simulink model "mainModel"  (R2025a)
settings: Solver=VariableStepAuto  StartTime=0  StopTime=5000  RelTol=1e-3
values from neighbouring files (symbols this model uses):
  advectiveCoefficientScale = 400    [constant_parameters.m]    (also in runScript.m = 100)
  AmbientTemperature = out{4}    [runScript.m]
  massCoolantScale = 0.01    [constant_parameters.m]    (also in runScript.m = 0.003)
  massModuleScale = 11    [constant_parameters.m]    (also in runScript.m)
  scaledAdvectiveCoefficient = 1.2    [runScript.m]
  scaledMassCoolant = 0.8    [runScript.m]
  scaledMassModule = 1.2    [runScript.m]
libraries: fl_lib x231, coolantFlow_lib x65, nesl_utility x35, IONIQ_parameters2_lib x32, algebraicManip_lib x32, batt_lib x1
settings Model: Creator=mbhattu  LastModifiedBy=mbhattu
settings SimscapeCC: SimscapeLogType=all

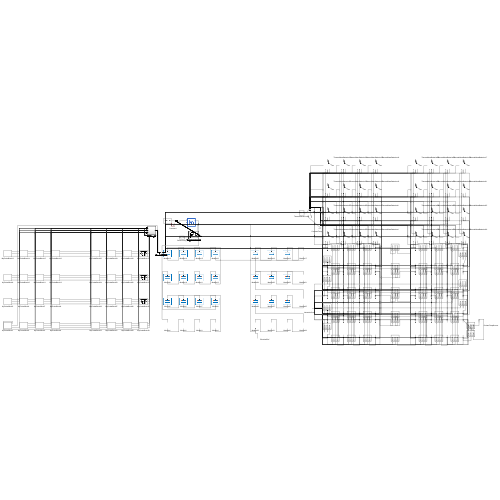
[thumbnail: Simulink's stored preview of the top-level diagram]
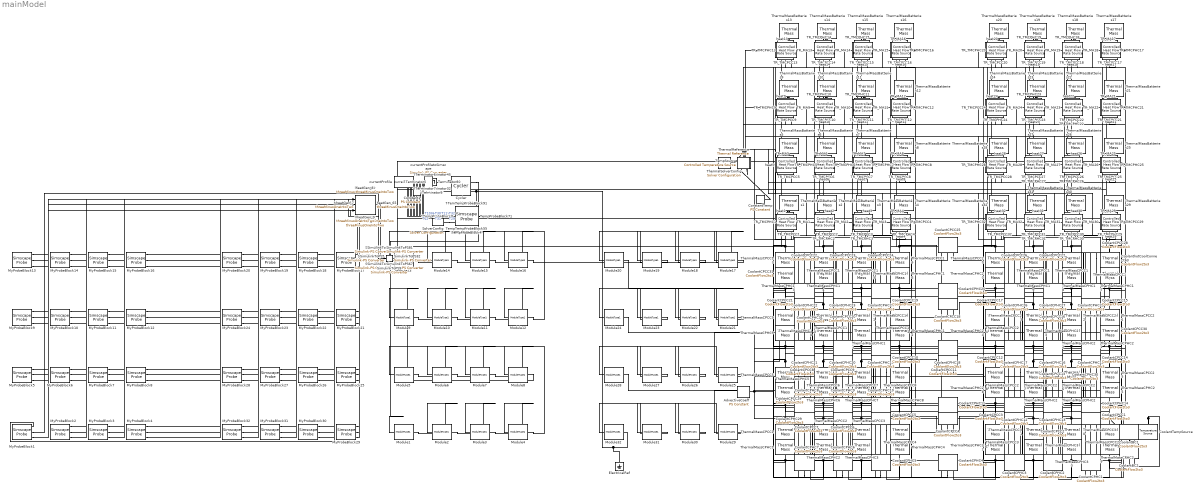
== system mainModel ==
  AdvectiveCoeff : fl_lib/Physical Signals/Sources/PS Constant  constant=advectiveCoefficientScale * scaledAdvectiveCoefficient W/K
  Constant1 : fl_lib/Physical Signals/Sources/PS Constant  constant=1
  ConstantTemp : fl_lib/Physical Signals/Sources/PS Constant  constant=AmbientTemperature
  CoolantBC1 : coolantFlow_lib/CoolantFlow2to3  SystemSampleTime=-1  VariantActivationTime=update diagram  EmptyChoice=off  PassThrough=off  PassThroughVariantControl=(default)  EmptyChoiceVariantControl=(default)  AllowFlexibleInterface=on  Latency=0  AutoFrameSizeCalculation=off
  CoolantBC2 : coolantFlow_lib/CoolantFlow2to3  SystemSampleTime=-1  VariantActivationTime=update diagram  EmptyChoice=off  PassThrough=off  PassThroughVariantControl=(default)  EmptyChoiceVariantControl=(default)  AllowFlexibleInterface=on  Latency=0  AutoFrameSizeCalculation=off
  CoolantCPCC{1..31} (31 alike) : coolantFlow_lib/CoolantFlow2to3  SystemSampleTime=-1  VariantActivationTime=update diagram  EmptyChoice=off  PassThrough=off  PassThroughVariantControl=(default)  EmptyChoiceVariantControl=(default)  AllowFlexibleInterface=on  Latency=0  AutoFrameSizeCalculation=off
  CoolantCPHC{1..31} (31 alike) : coolantFlow_lib/CoolantFlow2to3  SystemSampleTime=-1  VariantActivationTime=update diagram  EmptyChoice=off  PassThrough=off  PassThroughVariantControl=(default)  EmptyChoiceVariantControl=(default)  AllowFlexibleInterface=on  Latency=0  AutoFrameSizeCalculation=off
  CoolantTempSource : fl_lib/Thermal/Thermal Sources/Temperature Source  temperature=coolantTempSourceTemperature K
  CoolanthotCoolConnect63 : coolantFlow_lib/CoolantFlow2to3  SystemSampleTime=-1  VariantActivationTime=update diagram  EmptyChoice=off  PassThrough=off  PassThroughVariantControl=(default)  EmptyChoiceVariantControl=(default)  AllowFlexibleInterface=on  Latency=0  AutoFrameSizeCalculation=off
  Cycler : batt_lib/Cyclers/Cycler  current_option=simscape.battery.enum.cyclers.positive_current.Discharge  configuration_option=simscape.battery.enum.cyclers.device_configuration.Cycler
      settings: InternalSimscapePortConfiguration="{\"Bottom\":[],\"Left\":[{\"id\":\"iT\",\"label\":\"i\",\"type\":\"input\"},{\"id\":\"vT\",\"label\":\"v\",\"type\":\"input\"},{\"id\":\"c\",\"label\":\"c\",\"type\":\"input\"}],\"Right\":[{\"id\":\"p\",\"label\":\"+\",\"type\":\"foundation.electrical.electrical\"},{\"id\":\"n\",\"label\":\"-\",\"type\":\"foundation.electrical.electrical\"}],\"Top\":[]}"
  ElectricalRef : fl_lib/Electrical/Electrical Elements/Electrical Reference
  Module{1..32} (32 alike) : IONIQ_parameters2_lib/Modules/ModuleType1  BatteryCapacityCell=ModuleType1.BatteryCapacityCell A*hr  ExtrapolationMethodCell=simscape.enum.extrapolation.nearest  SOCBreakpointsCell=ModuleType1.SOCBreakpointsCell  TemperatureBreakpointsCell=ModuleType1.TemperatureBreakpointsCell K  OpenCircuitVoltageThermalCell=ModuleType1.OpenCircuitVoltageThermalCell V  VoltageRangeCell=ModuleType1.VoltageRangeCell V  ResistanceSOCBreakpointsCell=ModuleType1.ResistanceSOCBreakpointsCell  ResistanceTemperatureBreakpointsCell=ModuleType1.ResistanceTemperatureBreakpointsCell K  R0ThermalCell=ModuleType1.R0ThermalCell Ohm  R1ThermalCell=ModuleType1.R1ThermalCell Ohm  Tau1ThermalCell=ModuleType1.Tau1ThermalCell s  SimulationTemperatureCell=ModuleType1.SimulationTemperatureCell K  P=2  S=6  socCell_specify=on  socCell_priority=High  socCell=Module1.socCell  socCell_nominal_specify=off  socCell_nominal_value=1  socCell_nominal_unit=1  batteryVoltage_specify=on  batteryVoltage_priority=None  batteryVoltage=Module1.batteryVoltage V  batteryVoltage_nominal_specify=off  batteryVoltage_nominal_value=1  batteryVoltage_nominal_unit=V  batteryCurrent_specify=on  batteryCurrent_priority=None  batteryCurrent=Module1.batteryCurrent A  batteryCurrent_nominal_specify=off  batteryCurrent_nominal_value=1  batteryCurrent_nominal_unit=A  numCycles_specify=on  numCycles_priority=High  numCycles=Module1.numCycles  numCycles_nominal_specify=off  numCycles_nominal_value=1  numCycles_nominal_unit=1  vParallelAssembly_specify=on  vParallelAssembly_priority=None  vParallelAssembly=Module1.vParallelAssembly V  vParallelAssembly_nominal_specify=off  vParallelAssembly_nominal_value=1  vParallelAssembly_nominal_unit=V  socParallelAssembly_specify=on  socParallelAssembly_priority=None  socParallelAssembly=Module1.socParallelAssembly  socParallelAssembly_nominal_specify=off  socParallelAssembly_nominal_value=1  socParallelAssembly_nominal_unit=1
      settings: InternalSimscapePortConfiguration="{\"Bottom\":[{\"id\":\"n\",\"label\":\"-\",\"type\":\"foundation.electrical.electrical\"}],\"Left\":[],\"Right\":[],\"Top\":[{\"id\":\"p\",\"label\":\"+\",\"type\":\"foundation.electrical.electrical\"}]}"
  MyProbeBlock1 : SimscapeProbe  BoundBlock=1  Variables="{\"Cell1.batteryCurrent\":{\"Probing\":\"ON\"},\"Cell1.batteryVoltage\":{\"Probing\":\"ON\"},\"Cell1.ocv\":{\"Probing\":\"ON\"}}"
  MyProbeBlock10 : SimscapeProbe  BoundBlock=10  Variables="{\"Cell1.batteryCurrent\":{\"Probing\":\"ON\"},\"Cell1.batteryVoltage\":{\"Probing\":\"ON\"},\"Cell1.ocv\":{\"Probing\":\"ON\"}}"
  MyProbeBlock11 : SimscapeProbe  BoundBlock=11  Variables="{\"Cell1.batteryCurrent\":{\"Probing\":\"ON\"},\"Cell1.batteryVoltage\":{\"Probing\":\"ON\"},\"Cell1.ocv\":{\"Probing\":\"ON\"}}"
  MyProbeBlock12 : SimscapeProbe  BoundBlock=12  Variables="{\"Cell1.batteryCurrent\":{\"Probing\":\"ON\"},\"Cell1.batteryVoltage\":{\"Probing\":\"ON\"},\"Cell1.ocv\":{\"Probing\":\"ON\"}}"
  MyProbeBlock13 : SimscapeProbe  BoundBlock=13  Variables="{\"Cell1.batteryCurrent\":{\"Probing\":\"ON\"},\"Cell1.batteryVoltage\":{\"Probing\":\"ON\"},\"Cell1.ocv\":{\"Probing\":\"ON\"}}"
  MyProbeBlock14 : SimscapeProbe  BoundBlock=14  Variables="{\"Cell1.batteryCurrent\":{\"Probing\":\"ON\"},\"Cell1.batteryVoltage\":{\"Probing\":\"ON\"},\"Cell1.ocv\":{\"Probing\":\"ON\"}}"
  MyProbeBlock15 : SimscapeProbe  BoundBlock=15  Variables="{\"Cell1.batteryCurrent\":{\"Probing\":\"ON\"},\"Cell1.batteryVoltage\":{\"Probing\":\"ON\"},\"Cell1.ocv\":{\"Probing\":\"ON\"}}"
  MyProbeBlock16 : SimscapeProbe  BoundBlock=16  Variables="{\"Cell1.batteryCurrent\":{\"Probing\":\"ON\"},\"Cell1.batteryVoltage\":{\"Probing\":\"ON\"},\"Cell1.ocv\":{\"Probing\":\"ON\"}}"
  MyProbeBlock17 : SimscapeProbe  BoundBlock=17  Variables="{\"Cell1.batteryCurrent\":{\"Probing\":\"ON\"},\"Cell1.batteryVoltage\":{\"Probing\":\"ON\"},\"Cell1.ocv\":{\"Probing\":\"ON\"}}"
  MyProbeBlock18 : SimscapeProbe  BoundBlock=18  Variables="{\"Cell1.batteryCurrent\":{\"Probing\":\"ON\"},\"Cell1.batteryVoltage\":{\"Probing\":\"ON\"},\"Cell1.ocv\":{\"Probing\":\"ON\"}}"
  MyProbeBlock19 : SimscapeProbe  BoundBlock=19  Variables="{\"Cell1.batteryCurrent\":{\"Probing\":\"ON\"},\"Cell1.batteryVoltage\":{\"Probing\":\"ON\"},\"Cell1.ocv\":{\"Probing\":\"ON\"}}"
  MyProbeBlock2 : SimscapeProbe  BoundBlock=2  Variables="{\"Cell1.batteryCurrent\":{\"Probing\":\"ON\"},\"Cell1.batteryVoltage\":{\"Probing\":\"ON\"},\"Cell1.ocv\":{\"Probing\":\"ON\"}}"
  MyProbeBlock20 : SimscapeProbe  BoundBlock=20  Variables="{\"Cell1.batteryCurrent\":{\"Probing\":\"ON\"},\"Cell1.batteryVoltage\":{\"Probing\":\"ON\"},\"Cell1.ocv\":{\"Probing\":\"ON\"}}"
  MyProbeBlock21 : SimscapeProbe  BoundBlock=21  Variables="{\"Cell1.batteryCurrent\":{\"Probing\":\"ON\"},\"Cell1.batteryVoltage\":{\"Probing\":\"ON\"},\"Cell1.ocv\":{\"Probing\":\"ON\"}}"
  MyProbeBlock22 : SimscapeProbe  BoundBlock=22  Variables="{\"Cell1.batteryCurrent\":{\"Probing\":\"ON\"},\"Cell1.batteryVoltage\":{\"Probing\":\"ON\"},\"Cell1.ocv\":{\"Probing\":\"ON\"}}"
  MyProbeBlock23 : SimscapeProbe  BoundBlock=23  Variables="{\"Cell1.batteryCurrent\":{\"Probing\":\"ON\"},\"Cell1.batteryVoltage\":{\"Probing\":\"ON\"},\"Cell1.ocv\":{\"Probing\":\"ON\"}}"
  MyProbeBlock24 : SimscapeProbe  BoundBlock=24  Variables="{\"Cell1.batteryCurrent\":{\"Probing\":\"ON\"},\"Cell1.batteryVoltage\":{\"Probing\":\"ON\"},\"Cell1.ocv\":{\"Probing\":\"ON\"}}"
  MyProbeBlock25 : SimscapeProbe  BoundBlock=25  Variables="{\"Cell1.batteryCurrent\":{\"Probing\":\"ON\"},\"Cell1.batteryVoltage\":{\"Probing\":\"ON\"},\"Cell1.ocv\":{\"Probing\":\"ON\"}}"
  MyProbeBlock26 : SimscapeProbe  BoundBlock=26  Variables="{\"Cell1.batteryCurrent\":{\"Probing\":\"ON\"},\"Cell1.batteryVoltage\":{\"Probing\":\"ON\"},\"Cell1.ocv\":{\"Probing\":\"ON\"}}"
  MyProbeBlock27 : SimscapeProbe  BoundBlock=27  Variables="{\"Cell1.batteryCurrent\":{\"Probing\":\"ON\"},\"Cell1.batteryVoltage\":{\"Probing\":\"ON\"},\"Cell1.ocv\":{\"Probing\":\"ON\"}}"
  MyProbeBlock28 : SimscapeProbe  BoundBlock=28  Variables="{\"Cell1.batteryCurrent\":{\"Probing\":\"ON\"},\"Cell1.batteryVoltage\":{\"Probing\":\"ON\"},\"Cell1.ocv\":{\"Probing\":\"ON\"}}"
  MyProbeBlock29 : SimscapeProbe  BoundBlock=29  Variables="{\"Cell1.batteryCurrent\":{\"Probing\":\"ON\"},\"Cell1.batteryVoltage\":{\"Probing\":\"ON\"},\"Cell1.ocv\":{\"Probing\":\"ON\"}}"
  MyProbeBlock3 : SimscapeProbe  BoundBlock=3  Variables="{\"Cell1.batteryCurrent\":{\"Probing\":\"ON\"},\"Cell1.batteryVoltage\":{\"Probing\":\"ON\"},\"Cell1.ocv\":{\"Probing\":\"ON\"}}"
  MyProbeBlock30 : SimscapeProbe  BoundBlock=30  Variables="{\"Cell1.batteryCurrent\":{\"Probing\":\"ON\"},\"Cell1.batteryVoltage\":{\"Probing\":\"ON\"},\"Cell1.ocv\":{\"Probing\":\"ON\"}}"
  MyProbeBlock31 : SimscapeProbe  BoundBlock=31  Variables="{\"Cell1.batteryCurrent\":{\"Probing\":\"ON\"},\"Cell1.batteryVoltage\":{\"Probing\":\"ON\"},\"Cell1.ocv\":{\"Probing\":\"ON\"}}"
  MyProbeBlock32 : SimscapeProbe  BoundBlock=32  Variables="{\"Cell1.batteryCurrent\":{\"Probing\":\"ON\"},\"Cell1.batteryVoltage\":{\"Probing\":\"ON\"},\"Cell1.ocv\":{\"Probing\":\"ON\"}}"
  MyProbeBlock4 : SimscapeProbe  BoundBlock=4  Variables="{\"Cell1.batteryCurrent\":{\"Probing\":\"ON\"},\"Cell1.batteryVoltage\":{\"Probing\":\"ON\"},\"Cell1.ocv\":{\"Probing\":\"ON\"}}"
  MyProbeBlock5 : SimscapeProbe  BoundBlock=5  Variables="{\"Cell1.batteryCurrent\":{\"Probing\":\"ON\"},\"Cell1.batteryVoltage\":{\"Probing\":\"ON\"},\"Cell1.ocv\":{\"Probing\":\"ON\"}}"
  MyProbeBlock6 : SimscapeProbe  BoundBlock=6  Variables="{\"Cell1.batteryCurrent\":{\"Probing\":\"ON\"},\"Cell1.batteryVoltage\":{\"Probing\":\"ON\"},\"Cell1.ocv\":{\"Probing\":\"ON\"}}"
  MyProbeBlock7 : SimscapeProbe  BoundBlock=7  Variables="{\"Cell1.batteryCurrent\":{\"Probing\":\"ON\"},\"Cell1.batteryVoltage\":{\"Probing\":\"ON\"},\"Cell1.ocv\":{\"Probing\":\"ON\"}}"
  MyProbeBlock8 : SimscapeProbe  BoundBlock=8  Variables="{\"Cell1.batteryCurrent\":{\"Probing\":\"ON\"},\"Cell1.batteryVoltage\":{\"Probing\":\"ON\"},\"Cell1.ocv\":{\"Probing\":\"ON\"}}"
  MyProbeBlock9 : SimscapeProbe  BoundBlock=9  Variables="{\"Cell1.batteryCurrent\":{\"Probing\":\"ON\"},\"Cell1.batteryVoltage\":{\"Probing\":\"ON\"},\"Cell1.ocv\":{\"Probing\":\"ON\"}}"
  SimulinkToPS{1..32} (32 alike) : nesl_utility/Simulink-PS Converter  PhysicalDomain=network_engine_domain  SubClassName=ps_input  LeftPortType=input  RightPortType=output  PseudoPeriodic=off  Frequencies=[]  NoiseDistribution=none  NoiseParameters=[]  Unit=1  AffineConversion=off  FilteringAndDerivatives=provide  SimscapeFilterOrder=1  InputFilterTimeConstant=0.001  UdotUserProvided=0
  SolverConfig : nesl_utility/Solver Configuration  PhysicalDomain=network_engine_domain  SubClassName=solver  LeftPortType=input  RightPortType=generic  Tones=[]  Harmonics=[]  SimulateNoise=off  Profile=off  UseLocalSampling=off  EnableSwitchedLinearOptims=on  FrequencyDomain=off  UseCCode=off  RelTol=0.001  AbsTol=0.001  MinStep=1e-09  ToWorkspace=off  RevertToSquareIcSolve=off  NumHomotopyIterations=100  PhasorMode=off  PhasorModeNumHarmonics=1  ConsistencySolver=NEWTON_XTOL_AFTER_FTOL  IndexReductionMethod=DerivativeReplacement  DoDC=off  ResidualTolerance=1e-09  ConsistencyTolSource=GLOBAL  ConsistencyAbsTol=0.001  ConsistencyRelTol=0.001  ConsistencyTolFactor=0.001  UseLocalSolver=off  LocalSolverChoice=NE_BACKWARD_EULER_ADVANCER  ResolveIndetEquations=on  FunctionEvalNumThread=1  LocalSolverSampleTime=0.001  DoFixedCost=off  MaxNonlinIter=3  MaxModeIter=2  ComputeImpulses=off  ImpulseIterations=2  LinearAlgebra=auto  LinearAlgebraNumThread=0  EquationFormulation=NE_TIME_EF  DelaysMemoryBudget=1024  AutomaticFiltering=on  FilteringTimeConstant=0.001  PartitionStorageMethod=AS_NEEDED  PartitionMemoryBudget=1024  PartitionMethod=ROBUST  MultibodyUseLocalSolver=off  MultibodyLocalSolverChoice=ODE1  MultibodyLocalSolverSampleTime=0.001
  TR_MA{1,5,9,13,17,21,25,29} (8 alike) : fl_lib/Thermal/Thermal Elements/Thermal Resistance  resistance=thermalResistanceModuleToAmbient_1 K/W  T_specify=off  T_priority=None  T=0 K  T_nominal_specify=off  T_nominal_value=1  T_nominal_unit=K  Q_specify=off  Q_priority=None  Q=0 W  Q_nominal_specify=off  Q_nominal_value=1  Q_nominal_unit=W
  TR_MA{2,6,10,14,18,22,26,30} (8 alike) : fl_lib/Thermal/Thermal Elements/Thermal Resistance  resistance=thermalResistanceModuleToAmbient_2 K/W  T_specify=off  T_priority=None  T=0 K  T_nominal_specify=off  T_nominal_value=1  T_nominal_unit=K  Q_specify=off  Q_priority=None  Q=0 W  Q_nominal_specify=off  Q_nominal_value=1  Q_nominal_unit=W
  TR_MA{3,7,11,15,19,23,27,31} (8 alike) : fl_lib/Thermal/Thermal Elements/Thermal Resistance  resistance=thermalResistanceModuleToAmbient_3 K/W  T_specify=off  T_priority=None  T=0 K  T_nominal_specify=off  T_nominal_value=1  T_nominal_unit=K  Q_specify=off  Q_priority=None  Q=0 W  Q_nominal_specify=off  Q_nominal_value=1  Q_nominal_unit=W
  TR_MA{4,8,12,16,20,24,28,32} (8 alike) : fl_lib/Thermal/Thermal Elements/Thermal Resistance  resistance=thermalResistanceModuleToAmbient_0 K/W  T_specify=off  T_priority=None  T=0 K  T_nominal_specify=off  T_nominal_value=1  T_nominal_unit=K  Q_specify=off  Q_priority=None  Q=0 W  Q_nominal_specify=off  Q_nominal_value=1  Q_nominal_unit=W
  TR_TMCPCC{1..32} (32 alike) : fl_lib/Thermal/Thermal Elements/Thermal Resistance  resistance=thermalResistanceTubeToModule K/W  T_specify=off  T_priority=None  T=0 K  T_nominal_specify=off  T_nominal_value=1  T_nominal_unit=K  Q_specify=off  Q_priority=None  Q=0 W  Q_nominal_specify=off  Q_nominal_value=1  Q_nominal_unit=W
  TR_TMCPHC{1..32} (32 alike) : fl_lib/Thermal/Thermal Elements/Thermal Resistance  resistance=thermalResistanceTubeToModule K/W  T_specify=off  T_priority=None  T=0 K  T_nominal_specify=off  T_nominal_value=1  T_nominal_unit=K  Q_specify=off  Q_priority=None  Q=0 W  Q_nominal_specify=off  Q_nominal_value=1  Q_nominal_unit=W
  TempProbeBlock1 : SimscapeProbe  BoundBlock=135  Variables="{\"M.T\":{\"Probing\":\"ON\"}}"
  TempProbeBlock10 : SimscapeProbe  BoundBlock=144  Variables="{\"M.T\":{\"Probing\":\"ON\"}}"
  TempProbeBlock11 : SimscapeProbe  BoundBlock=145  Variables="{\"M.T\":{\"Probing\":\"ON\"}}"
  TempProbeBlock12 : SimscapeProbe  BoundBlock=146  Variables="{\"M.T\":{\"Probing\":\"ON\"}}"
  TempProbeBlock13 : SimscapeProbe  BoundBlock=147  Variables="{\"M.T\":{\"Probing\":\"ON\"}}"
  TempProbeBlock14 : SimscapeProbe  BoundBlock=148  Variables="{\"M.T\":{\"Probing\":\"ON\"}}"
  TempProbeBlock15 : SimscapeProbe  BoundBlock=149  Variables="{\"M.T\":{\"Probing\":\"ON\"}}"
  TempProbeBlock16 : SimscapeProbe  BoundBlock=150  Variables="{\"M.T\":{\"Probing\":\"ON\"}}"
  TempProbeBlock17 : SimscapeProbe  BoundBlock=151  Variables="{\"M.T\":{\"Probing\":\"ON\"}}"
  TempProbeBlock18 : SimscapeProbe  BoundBlock=152  Variables="{\"M.T\":{\"Probing\":\"ON\"}}"
  TempProbeBlock19 : SimscapeProbe  BoundBlock=153  Variables="{\"M.T\":{\"Probing\":\"ON\"}}"
  TempProbeBlock2 : SimscapeProbe  BoundBlock=136  Variables="{\"M.T\":{\"Probing\":\"ON\"}}"
  TempProbeBlock20 : SimscapeProbe  BoundBlock=154  Variables="{\"M.T\":{\"Probing\":\"ON\"}}"
  TempProbeBlock21 : SimscapeProbe  BoundBlock=155  Variables="{\"M.T\":{\"Probing\":\"ON\"}}"
  TempProbeBlock22 : SimscapeProbe  BoundBlock=156  Variables="{\"M.T\":{\"Probing\":\"ON\"}}"
  TempProbeBlock23 : SimscapeProbe  BoundBlock=157  Variables="{\"M.T\":{\"Probing\":\"ON\"}}"
  TempProbeBlock24 : SimscapeProbe  BoundBlock=158  Variables="{\"M.T\":{\"Probing\":\"ON\"}}"
  TempProbeBlock25 : SimscapeProbe  BoundBlock=159  Variables="{\"M.T\":{\"Probing\":\"ON\"}}"
  TempProbeBlock26 : SimscapeProbe  BoundBlock=160  Variables="{\"M.T\":{\"Probing\":\"ON\"}}"
  TempProbeBlock27 : SimscapeProbe  BoundBlock=161  Variables="{\"M.T\":{\"Probing\":\"ON\"}}"
  TempProbeBlock28 : SimscapeProbe  BoundBlock=162  Variables="{\"M.T\":{\"Probing\":\"ON\"}}"
  TempProbeBlock29 : SimscapeProbe  BoundBlock=163  Variables="{\"M.T\":{\"Probing\":\"ON\"}}"
  TempProbeBlock3 : SimscapeProbe  BoundBlock=137  Variables="{\"M.T\":{\"Probing\":\"ON\"}}"
  TempProbeBlock30 : SimscapeProbe  BoundBlock=164  Variables="{\"M.T\":{\"Probing\":\"ON\"}}"
  TempProbeBlock31 : SimscapeProbe  BoundBlock=165  Variables="{\"M.T\":{\"Probing\":\"ON\"}}"
  TempProbeBlock32 : SimscapeProbe  BoundBlock=166  Variables="{\"M.T\":{\"Probing\":\"ON\"}}"
  TempProbeBlock4 : SimscapeProbe  BoundBlock=138  Variables="{\"M.T\":{\"Probing\":\"ON\"}}"
  TempProbeBlock5 : SimscapeProbe  BoundBlock=139  Variables="{\"M.T\":{\"Probing\":\"ON\"}}"
  TempProbeBlock6 : SimscapeProbe  BoundBlock=140  Variables="{\"M.T\":{\"Probing\":\"ON\"}}"
  TempProbeBlock7 : SimscapeProbe  BoundBlock=141  Variables="{\"M.T\":{\"Probing\":\"ON\"}}"
  TempProbeBlock8 : SimscapeProbe  BoundBlock=142  Variables="{\"M.T\":{\"Probing\":\"ON\"}}"
  TempProbeBlock9 : SimscapeProbe  BoundBlock=143  Variables="{\"M.T\":{\"Probing\":\"ON\"}}"
  TempSource : fl_lib/Thermal/Thermal Sources/Controlled Temperature Source
  Terminator{1..32} (32 alike) : Terminator
  ThermalMassBatteries{1..32} (32 alike) : fl_lib/Thermal/Thermal Elements/Thermal Mass  mass_type=foundation.enum.constant_variable.constant  mass=massModuleScale * scaledMassModule kg  sp_heat=CpModule J/(K*kg)  mass_min=1e-6 kg  num_ports=foundation.enum.numPorts2.one  m_specify=off  m_priority=High  m=1 kg  m_nominal_specify=off  m_nominal_value=1  m_nominal_unit=kg  T_specify=on  T_priority=High  T=AmbientTemperature K  T_nominal_specify=off  T_nominal_value=1  T_nominal_unit=K  Q_specify=off  Q_priority=None  Q=0 W  Q_nominal_specify=off  Q_nominal_value=1  Q_nominal_unit=W
  ThermalMassCPCC{1..32} (32 alike) : fl_lib/Thermal/Thermal Elements/Thermal Mass  mass_type=foundation.enum.constant_variable.constant  mass=massCoolantScale * scaledMassCoolant kg  sp_heat=CpCoolant J/(K*kg)  mass_min=1e-6 kg  num_ports=foundation.enum.numPorts2.one  m_specify=off  m_priority=High  m=1 kg  m_nominal_specify=off  m_nominal_value=1  m_nominal_unit=kg  T_specify=on  T_priority=High  T=AmbientTemperature K  T_nominal_specify=off  T_nominal_value=1  T_nominal_unit=K  Q_specify=off  Q_priority=None  Q=0 W  Q_nominal_specify=off  Q_nominal_value=1  Q_nominal_unit=W
  ThermalMassCPHC{1..32} (32 alike) : fl_lib/Thermal/Thermal Elements/Thermal Mass  mass_type=foundation.enum.constant_variable.constant  mass=massCoolantScale * scaledMassCoolant kg  sp_heat=CpCoolant J/(K*kg)  mass_min=1e-6 kg  num_ports=foundation.enum.numPorts2.one  m_specify=off  m_priority=High  m=1 kg  m_nominal_specify=off  m_nominal_value=1  m_nominal_unit=kg  T_specify=on  T_priority=High  T=AmbientTemperature K  T_nominal_specify=off  T_nominal_value=1  T_nominal_unit=K  Q_specify=off  Q_priority=None  Q=0 W  Q_nominal_specify=off  Q_nominal_value=1  Q_nominal_unit=W
  ThermalReference : fl_lib/Thermal/Thermal Elements/Thermal Reference
  ThermalSolverConfig : nesl_utility/Solver Configuration  PhysicalDomain=network_engine_domain  SubClassName=solver  LeftPortType=input  RightPortType=generic  Tones=[]  Harmonics=[]  SimulateNoise=off  Profile=off  UseLocalSampling=off  EnableSwitchedLinearOptims=on  FrequencyDomain=off  UseCCode=off  RelTol=0.001  AbsTol=0.001  MinStep=1e-09  ToWorkspace=off  RevertToSquareIcSolve=off  NumHomotopyIterations=100  PhasorMode=off  PhasorModeNumHarmonics=1  ConsistencySolver=NEWTON_XTOL_AFTER_FTOL  IndexReductionMethod=DerivativeReplacement  DoDC=off  ResidualTolerance=1e-09  ConsistencyTolSource=GLOBAL  ConsistencyAbsTol=0.001  ConsistencyRelTol=0.001  ConsistencyTolFactor=0.001  UseLocalSolver=off  LocalSolverChoice=NE_BACKWARD_EULER_ADVANCER  ResolveIndetEquations=on  FunctionEvalNumThread=1  LocalSolverSampleTime=0.001  DoFixedCost=off  MaxNonlinIter=3  MaxModeIter=2  ComputeImpulses=off  ImpulseIterations=2  LinearAlgebra=auto  LinearAlgebraNumThread=0  EquationFormulation=NE_TIME_EF  DelaysMemoryBudget=1024  AutomaticFiltering=on  FilteringTimeConstant=0.001  PartitionStorageMethod=AS_NEEDED  PartitionMemoryBudget=1024  PartitionMethod=ROBUST  MultibodyUseLocalSolver=off  MultibodyLocalSolverChoice=ODE1  MultibodyLocalSolverSampleTime=0.001
  currentProfile : FromWorkspace  VariableName=currentData
  currentProfiletoSimscape : nesl_utility/Simulink-PS Converter  PhysicalDomain=network_engine_domain  SubClassName=ps_input  LeftPortType=input  RightPortType=output  PseudoPeriodic=off  Frequencies=[]  NoiseDistribution=none  NoiseParameters=[]  Unit=1  AffineConversion=off  FilteringAndDerivatives=provide  SimscapeFilterOrder=1  InputFilterTimeConstant=0.001  UdotUserProvided=0
  heat{1..32} (32 alike) : fl_lib/Thermal/Thermal Sources/Controlled Heat Flow Rate Source
  heatGen_{1..32} (32 alike) : algebraicManip_lib/threeMinusOneIntoTwo  SystemSampleTime=-1  VariantActivationTime=update diagram  EmptyChoice=off  PassThrough=off  PassThroughVariantControl=(default)  EmptyChoiceVariantControl=(default)  AllowFlexibleInterface=on  Latency=0  AutoFrameSizeCalculation=off
  wires:
  currentProfile/1 -> currentProfiletoSimscape/1
  MyProbeBlock1/3 -> heatGen_1/1
  MyProbeBlock1/1 -> heatGen_1/2
  MyProbeBlock1/2 -> heatGen_1/3
  heatGen_1/1 -> SimulinkToPS1/1
  MyProbeBlock2/3 -> heatGen_2/1
  MyProbeBlock2/1 -> heatGen_2/2
  MyProbeBlock2/2 -> heatGen_2/3
  heatGen_2/1 -> SimulinkToPS2/1
  MyProbeBlock3/3 -> heatGen_3/1
  MyProbeBlock3/1 -> heatGen_3/2
  MyProbeBlock3/2 -> heatGen_3/3
  heatGen_3/1 -> SimulinkToPS3/1
  MyProbeBlock4/3 -> heatGen_4/1
  MyProbeBlock4/1 -> heatGen_4/2
  MyProbeBlock4/2 -> heatGen_4/3
  heatGen_4/1 -> SimulinkToPS4/1
  MyProbeBlock5/3 -> heatGen_5/1
  MyProbeBlock5/1 -> heatGen_5/2
  MyProbeBlock5/2 -> heatGen_5/3
  heatGen_5/1 -> SimulinkToPS5/1
  MyProbeBlock6/3 -> heatGen_6/1
  MyProbeBlock6/1 -> heatGen_6/2
  MyProbeBlock6/2 -> heatGen_6/3
  heatGen_6/1 -> SimulinkToPS6/1
  MyProbeBlock7/3 -> heatGen_7/1
  MyProbeBlock7/1 -> heatGen_7/2
  MyProbeBlock7/2 -> heatGen_7/3
  heatGen_7/1 -> SimulinkToPS7/1
  MyProbeBlock8/3 -> heatGen_8/1
  MyProbeBlock8/1 -> heatGen_8/2
  MyProbeBlock8/2 -> heatGen_8/3
  heatGen_8/1 -> SimulinkToPS8/1
  MyProbeBlock9/3 -> heatGen_9/1
  MyProbeBlock9/1 -> heatGen_9/2
  MyProbeBlock9/2 -> heatGen_9/3
  heatGen_9/1 -> SimulinkToPS9/1
  MyProbeBlock10/3 -> heatGen_10/1
  MyProbeBlock10/1 -> heatGen_10/2
  MyProbeBlock10/2 -> heatGen_10/3
  heatGen_10/1 -> SimulinkToPS10/1
  MyProbeBlock11/3 -> heatGen_11/1
  MyProbeBlock11/1 -> heatGen_11/2
  MyProbeBlock11/2 -> heatGen_11/3
  heatGen_11/1 -> SimulinkToPS11/1
  MyProbeBlock12/3 -> heatGen_12/1
  MyProbeBlock12/1 -> heatGen_12/2
  MyProbeBlock12/2 -> heatGen_12/3
  heatGen_12/1 -> SimulinkToPS12/1
  MyProbeBlock13/3 -> heatGen_13/1
  MyProbeBlock13/1 -> heatGen_13/2
  MyProbeBlock13/2 -> heatGen_13/3
  heatGen_13/1 -> SimulinkToPS13/1
  MyProbeBlock14/3 -> heatGen_14/1
  MyProbeBlock14/1 -> heatGen_14/2
  MyProbeBlock14/2 -> heatGen_14/3
  heatGen_14/1 -> SimulinkToPS14/1
  MyProbeBlock15/3 -> heatGen_15/1
  MyProbeBlock15/1 -> heatGen_15/2
  MyProbeBlock15/2 -> heatGen_15/3
  heatGen_15/1 -> SimulinkToPS15/1
  MyProbeBlock16/3 -> heatGen_16/1
  MyProbeBlock16/1 -> heatGen_16/2
  MyProbeBlock16/2 -> heatGen_16/3
  heatGen_16/1 -> SimulinkToPS16/1
  MyProbeBlock17/3 -> heatGen_17/1
  MyProbeBlock17/1 -> heatGen_17/2
  MyProbeBlock17/2 -> heatGen_17/3
  heatGen_17/1 -> SimulinkToPS17/1
  MyProbeBlock18/3 -> heatGen_18/1
  MyProbeBlock18/1 -> heatGen_18/2
  MyProbeBlock18/2 -> heatGen_18/3
  heatGen_18/1 -> SimulinkToPS18/1
  MyProbeBlock19/3 -> heatGen_19/1
  MyProbeBlock19/1 -> heatGen_19/2
  MyProbeBlock19/2 -> heatGen_19/3
  heatGen_19/1 -> SimulinkToPS19/1
  MyProbeBlock20/3 -> heatGen_20/1
  MyProbeBlock20/1 -> heatGen_20/2
  MyProbeBlock20/2 -> heatGen_20/3
  heatGen_20/1 -> SimulinkToPS20/1
  MyProbeBlock21/3 -> heatGen_21/1
  MyProbeBlock21/1 -> heatGen_21/2
  MyProbeBlock21/2 -> heatGen_21/3
  heatGen_21/1 -> SimulinkToPS21/1
  MyProbeBlock22/3 -> heatGen_22/1
  MyProbeBlock22/1 -> heatGen_22/2
  MyProbeBlock22/2 -> heatGen_22/3
  heatGen_22/1 -> SimulinkToPS22/1
  MyProbeBlock23/3 -> heatGen_23/1
  MyProbeBlock23/1 -> heatGen_23/2
  MyProbeBlock23/2 -> heatGen_23/3
  heatGen_23/1 -> SimulinkToPS23/1
  MyProbeBlock24/3 -> heatGen_24/1
  MyProbeBlock24/1 -> heatGen_24/2
  MyProbeBlock24/2 -> heatGen_24/3
  heatGen_24/1 -> SimulinkToPS24/1
  MyProbeBlock25/3 -> heatGen_25/1
  MyProbeBlock25/1 -> heatGen_25/2
  MyProbeBlock25/2 -> heatGen_25/3
  heatGen_25/1 -> SimulinkToPS25/1
  MyProbeBlock26/3 -> heatGen_26/1
  MyProbeBlock26/1 -> heatGen_26/2
  MyProbeBlock26/2 -> heatGen_26/3
  heatGen_26/1 -> SimulinkToPS26/1
  MyProbeBlock27/3 -> heatGen_27/1
  MyProbeBlock27/1 -> heatGen_27/2
  MyProbeBlock27/2 -> heatGen_27/3
  heatGen_27/1 -> SimulinkToPS27/1
  MyProbeBlock28/3 -> heatGen_28/1
  MyProbeBlock28/1 -> heatGen_28/2
  MyProbeBlock28/2 -> heatGen_28/3
  heatGen_28/1 -> SimulinkToPS28/1
  MyProbeBlock29/3 -> heatGen_29/1
  MyProbeBlock29/1 -> heatGen_29/2
  MyProbeBlock29/2 -> heatGen_29/3
  heatGen_29/1 -> SimulinkToPS29/1
  MyProbeBlock30/3 -> heatGen_30/1
  MyProbeBlock30/1 -> heatGen_30/2
  MyProbeBlock30/2 -> heatGen_30/3
  heatGen_30/1 -> SimulinkToPS30/1
  MyProbeBlock31/3 -> heatGen_31/1
  MyProbeBlock31/1 -> heatGen_31/2
  MyProbeBlock31/2 -> heatGen_31/3
  heatGen_31/1 -> SimulinkToPS31/1
  MyProbeBlock32/3 -> heatGen_32/1
  MyProbeBlock32/1 -> heatGen_32/2
  MyProbeBlock32/2 -> heatGen_32/3
  heatGen_32/1 -> SimulinkToPS32/1
  TempProbeBlock1/1 -> Terminator1/1  "T1"
  TempProbeBlock2/1 -> Terminator2/1  "T2"
  TempProbeBlock3/1 -> Terminator3/1  "T3"
  TempProbeBlock4/1 -> Terminator4/1  "T4"
  TempProbeBlock5/1 -> Terminator5/1  "T5"
  TempProbeBlock6/1 -> Terminator6/1  "T6"
  TempProbeBlock7/1 -> Terminator7/1  "T7"
  TempProbeBlock8/1 -> Terminator8/1  "T8"
  TempProbeBlock9/1 -> Terminator9/1  "T9"
  TempProbeBlock10/1 -> Terminator10/1  "T10"
  TempProbeBlock11/1 -> Terminator11/1  "T11"
  TempProbeBlock12/1 -> Terminator12/1  "T12"
  TempProbeBlock13/1 -> Terminator13/1  "T13"
  TempProbeBlock14/1 -> Terminator14/1  "T14"
  TempProbeBlock15/1 -> Terminator15/1  "T15"
  TempProbeBlock16/1 -> Terminator16/1  "T16"
  TempProbeBlock17/1 -> Terminator17/1  "T17"
  TempProbeBlock18/1 -> Terminator18/1  "T18"
  TempProbeBlock19/1 -> Terminator19/1  "T19"
  TempProbeBlock20/1 -> Terminator20/1  "T20"
  TempProbeBlock21/1 -> Terminator21/1  "T21"
  TempProbeBlock22/1 -> Terminator22/1  "T22"
  TempProbeBlock23/1 -> Terminator23/1  "T23"
  TempProbeBlock24/1 -> Terminator24/1  "T24"
  TempProbeBlock25/1 -> Terminator25/1  "T25"
  TempProbeBlock26/1 -> Terminator26/1  "T26"
  TempProbeBlock27/1 -> Terminator27/1  "T27"
  TempProbeBlock28/1 -> Terminator28/1  "T28"
  TempProbeBlock29/1 -> Terminator29/1  "T29"
  TempProbeBlock30/1 -> Terminator30/1  "T30"
  TempProbeBlock31/1 -> Terminator31/1  "T31"
  TempProbeBlock32/1 -> Terminator32/1  "T32"
  connections:
  Module1/RConn1 -- Module2/LConn1
  Module2/RConn1 -- Module3/LConn1
  Module3/RConn1 -- Module4/LConn1
  Module4/RConn1 -- Module5/LConn1
  Module5/RConn1 -- Module6/LConn1
  Module6/RConn1 -- Module7/LConn1
  Module7/RConn1 -- Module8/LConn1
  Module8/RConn1 -- Module9/LConn1
  Module9/RConn1 -- Module10/LConn1
  Module10/RConn1 -- Module11/LConn1
  Module11/RConn1 -- Module12/LConn1
  Module12/RConn1 -- Module13/LConn1
  Module13/RConn1 -- Module14/LConn1
  Module14/RConn1 -- Module15/LConn1
  Module15/RConn1 -- Module16/LConn1
  Module16/RConn1 -- Module17/LConn1
  Module17/RConn1 -- Module18/LConn1
  Module18/RConn1 -- Module19/LConn1
  Module19/RConn1 -- Module20/LConn1
  Module20/RConn1 -- Module21/LConn1
  Module21/RConn1 -- Module22/LConn1
  Module22/RConn1 -- Module23/LConn1
  Module23/RConn1 -- Module24/LConn1
  Module24/RConn1 -- Module25/LConn1
  Module25/RConn1 -- Module26/LConn1
  Module26/RConn1 -- Module27/LConn1
  Module27/RConn1 -- Module28/LConn1
  Module28/RConn1 -- Module29/LConn1
  Module29/RConn1 -- Module30/LConn1
  Module30/RConn1 -- Module31/LConn1
  Module31/RConn1 -- Module32/LConn1
  Constant1/RConn1 -- Cycler/LConn3
  currentProfiletoSimscape/RConn1 -- Cycler/LConn1
  Cycler/RConn1 -- Module1/LConn1
  Cycler/RConn2 -- SolverConfig/RConn1 -- Module32/RConn1 -- ElectricalRef/LConn1
  CoolantCPCC1/LConn2 -- ThermalMassCPCC29/LConn1 -- TR_TMCPCC29/LConn1 -- CoolantBC1/LConn3
  CoolantCPCC1/LConn3 -- CoolantCPCC2/LConn2 -- ThermalMassCPCC30/LConn1 -- TR_TMCPCC30/LConn1
  CoolantCPCC1/LConn1 -- AdvectiveCoeff/RConn1 -- CoolantCPCC2/LConn1 -- CoolantCPCC3/LConn1 -- CoolantCPCC4/LConn1 -- CoolantCPCC5/LConn1 -- CoolantCPCC6/LConn1 -- CoolantCPCC7/LConn1 -- CoolantCPCC8/LConn1 -- CoolantCPCC9/LConn1 -- CoolantCPCC10/LConn1 -- CoolantCPCC11/LConn1 -- CoolantCPCC12/LConn1 -- CoolantCPCC13/LConn1 -- CoolantCPCC14/LConn1 -- CoolantCPCC15/LConn1 -- CoolantCPCC16/LConn1 -- CoolantCPCC17/LConn1 -- CoolantCPCC18/LConn1 -- CoolantCPCC19/LConn1 -- CoolantCPCC20/LConn1 -- CoolantCPCC21/LConn1 -- CoolantCPCC22/LConn1 -- CoolantCPCC23/LConn1 -- CoolantCPCC24/LConn1 -- CoolantCPCC25/LConn1 -- CoolantCPCC26/LConn1 -- CoolantCPCC27/LConn1 -- CoolantCPCC28/LConn1 -- CoolantCPCC29/LConn1 -- CoolantCPCC30/LConn1 -- CoolantCPCC31/LConn1 -- CoolantCPHC1/LConn1 -- CoolantCPHC2/LConn1 -- CoolantCPHC3/LConn1 -- CoolantCPHC4/LConn1 -- CoolantCPHC5/LConn1 -- CoolantCPHC6/LConn1 -- CoolantCPHC7/LConn1 -- CoolantCPHC8/LConn1 -- CoolantCPHC9/LConn1 -- CoolantCPHC10/LConn1 -- CoolantCPHC11/LConn1 -- CoolantCPHC12/LConn1 -- CoolantCPHC13/LConn1 -- CoolantCPHC14/LConn1 -- CoolantCPHC15/LConn1 -- CoolantCPHC16/LConn1 -- CoolantCPHC17/LConn1 -- CoolantCPHC18/LConn1 -- CoolantCPHC19/LConn1 -- CoolantCPHC20/LConn1 -- CoolantCPHC21/LConn1 -- CoolantCPHC22/LConn1 -- CoolantCPHC23/LConn1 -- CoolantCPHC24/LConn1 -- CoolantCPHC25/LConn1 -- CoolantCPHC26/LConn1 -- CoolantCPHC27/LConn1 -- CoolantCPHC28/LConn1 -- CoolantCPHC29/LConn1 -- CoolantCPHC30/LConn1 -- CoolantCPHC31/LConn1 -- CoolanthotCoolConnect63/LConn1 -- CoolantBC1/LConn1 -- CoolantBC2/LConn1
  CoolantCPCC2/LConn3 -- CoolantCPCC3/LConn2 -- ThermalMassCPCC31/LConn1 -- TR_TMCPCC31/LConn1
  CoolantCPCC3/LConn3 -- CoolantCPCC4/LConn2 -- ThermalMassCPCC32/LConn1 -- TR_TMCPCC32/LConn1
  CoolantCPCC4/LConn3 -- CoolantCPCC5/LConn2 -- ThermalMassCPCC4/LConn1 -- TR_TMCPCC4/LConn1
  CoolantCPCC5/LConn3 -- CoolantCPCC6/LConn2 -- ThermalMassCPCC3/LConn1 -- TR_TMCPCC3/LConn1
  CoolantCPCC6/LConn3 -- CoolantCPCC7/LConn2 -- ThermalMassCPCC2/LConn1 -- TR_TMCPCC2/LConn1
  CoolantCPCC7/LConn3 -- CoolantCPCC29/LConn2 -- ThermalMassCPCC1/LConn1 -- TR_TMCPCC1/LConn1
  CoolantCPCC8/LConn2 -- ThermalMassCPCC5/LConn1 -- CoolantCPCC29/LConn3 -- TR_TMCPCC5/LConn1
  CoolantCPCC8/LConn3 -- CoolantCPCC9/LConn2 -- ThermalMassCPCC6/LConn1 -- TR_TMCPCC6/LConn1
  CoolantCPCC9/LConn3 -- CoolantCPCC10/LConn2 -- ThermalMassCPCC7/LConn1 -- TR_TMCPCC7/LConn1
  CoolantCPCC10/LConn3 -- CoolantCPCC11/LConn2 -- ThermalMassCPCC8/LConn1 -- TR_TMCPCC8/LConn1
  CoolantCPCC11/LConn3 -- CoolantCPCC12/LConn2 -- ThermalMassCPCC28/LConn1 -- TR_TMCPCC28/LConn1
  CoolantCPCC12/LConn3 -- CoolantCPCC13/LConn2 -- ThermalMassCPCC27/LConn1 -- TR_TMCPCC27/LConn1
  CoolantCPCC13/LConn3 -- CoolantCPCC14/LConn2 -- ThermalMassCPCC26/LConn1 -- TR_TMCPCC26/LConn1
  CoolantCPCC14/LConn3 -- CoolantCPCC30/LConn2 -- ThermalMassCPCC25/LConn1 -- TR_TMCPCC25/LConn1
  CoolantCPCC15/LConn2 -- ThermalMassCPCC21/LConn1 -- CoolantCPCC30/LConn3 -- TR_TMCPCC21/LConn1
  CoolantCPCC15/LConn3 -- CoolantCPCC16/LConn2 -- ThermalMassCPCC22/LConn1 -- TR_TMCPCC22/LConn1
  CoolantCPCC16/LConn3 -- CoolantCPCC17/LConn2 -- ThermalMassCPCC23/LConn1 -- TR_TMCPCC23/LConn1
  CoolantCPCC17/LConn3 -- CoolantCPCC18/LConn2 -- ThermalMassCPCC24/LConn1 -- TR_TMCPCC24/LConn1
  CoolantCPCC18/LConn3 -- CoolantCPCC19/LConn2 -- ThermalMassCPCC12/LConn1 -- TR_TMCPCC12/LConn1
  CoolantCPCC19/LConn3 -- CoolantCPCC20/LConn2 -- ThermalMassCPCC11/LConn1 -- TR_TMCPCC11/LConn1
  CoolantCPCC20/LConn3 -- CoolantCPCC21/LConn2 -- ThermalMassCPCC10/LConn1 -- TR_TMCPCC10/LConn1
  CoolantCPCC21/LConn3 -- CoolantCPCC31/LConn2 -- ThermalMassCPCC9/LConn1 -- TR_TMCPCC9/LConn1
  CoolantCPCC22/LConn2 -- ThermalMassCPCC13/LConn1 -- CoolantCPCC31/LConn3 -- TR_TMCPCC13/LConn1
  CoolantCPCC22/LConn3 -- CoolantCPCC23/LConn2 -- ThermalMassCPCC14/LConn1 -- TR_TMCPCC14/LConn1
  CoolantCPCC23/LConn3 -- CoolantCPCC24/LConn2 -- ThermalMassCPCC15/LConn1 -- TR_TMCPCC15/LConn1
  CoolantCPCC24/LConn3 -- CoolantCPCC25/LConn2 -- ThermalMassCPCC16/LConn1 -- TR_TMCPCC16/LConn1
  CoolantCPCC25/LConn3 -- CoolantCPCC26/LConn2 -- ThermalMassCPCC20/LConn1 -- TR_TMCPCC20/LConn1
  CoolantCPCC26/LConn3 -- CoolantCPCC27/LConn2 -- ThermalMassCPCC19/LConn1 -- TR_TMCPCC19/LConn1
  CoolantCPCC27/LConn3 -- CoolantCPCC28/LConn2 -- ThermalMassCPCC18/LConn1 -- TR_TMCPCC18/LConn1
  CoolantCPCC28/LConn3 -- CoolanthotCoolConnect63/LConn2 -- ThermalMassCPCC17/LConn1 -- TR_TMCPCC17/LConn1
  CoolantCPHC1/LConn3 -- ThermalMassCPHC29/LConn1 -- TR_TMCPHC29/LConn1 -- CoolantBC2/LConn2
  CoolantCPHC1/LConn2 -- CoolantCPHC2/LConn3 -- ThermalMassCPHC30/LConn1 -- TR_TMCPHC30/LConn1
  CoolantCPHC2/LConn2 -- CoolantCPHC3/LConn3 -- ThermalMassCPHC31/LConn1 -- TR_TMCPHC31/LConn1
  CoolantCPHC3/LConn2 -- CoolantCPHC4/LConn3 -- ThermalMassCPHC32/LConn1 -- TR_TMCPHC32/LConn1
  CoolantCPHC4/LConn2 -- CoolantCPHC5/LConn3 -- ThermalMassCPHC4/LConn1 -- TR_TMCPHC4/LConn1
  CoolantCPHC5/LConn2 -- CoolantCPHC6/LConn3 -- ThermalMassCPHC3/LConn1 -- TR_TMCPHC3/LConn1
  CoolantCPHC6/LConn2 -- CoolantCPHC7/LConn3 -- ThermalMassCPHC2/LConn1 -- TR_TMCPHC2/LConn1
  CoolantCPHC7/LConn2 -- CoolantCPHC29/LConn3 -- ThermalMassCPHC1/LConn1 -- TR_TMCPHC1/LConn1
  CoolantCPHC8/LConn3 -- ThermalMassCPHC5/LConn1 -- CoolantCPHC29/LConn2 -- TR_TMCPHC5/LConn1
  CoolantCPHC8/LConn2 -- CoolantCPHC9/LConn3 -- ThermalMassCPHC6/LConn1 -- TR_TMCPHC6/LConn1
  CoolantCPHC9/LConn2 -- CoolantCPHC10/LConn3 -- ThermalMassCPHC7/LConn1 -- TR_TMCPHC7/LConn1
  CoolantCPHC10/LConn2 -- CoolantCPHC11/LConn3 -- ThermalMassCPHC8/LConn1 -- TR_TMCPHC8/LConn1
  CoolantCPHC11/LConn2 -- CoolantCPHC12/LConn3 -- ThermalMassCPHC28/LConn1 -- TR_TMCPHC28/LConn1
  CoolantCPHC12/LConn2 -- CoolantCPHC13/LConn3 -- ThermalMassCPHC27/LConn1 -- TR_TMCPHC27/LConn1
  CoolantCPHC13/LConn2 -- CoolantCPHC14/LConn3 -- ThermalMassCPHC26/LConn1 -- TR_TMCPHC26/LConn1
  CoolantCPHC14/LConn2 -- CoolantCPHC30/LConn3 -- ThermalMassCPHC25/LConn1 -- TR_TMCPHC25/LConn1
  CoolantCPHC15/LConn3 -- ThermalMassCPHC21/LConn1 -- CoolantCPHC30/LConn2 -- TR_TMCPHC21/LConn1
  CoolantCPHC15/LConn2 -- CoolantCPHC16/LConn3 -- ThermalMassCPHC22/LConn1 -- TR_TMCPHC22/LConn1
  CoolantCPHC16/LConn2 -- CoolantCPHC17/LConn3 -- ThermalMassCPHC23/LConn1 -- TR_TMCPHC23/LConn1
  CoolantCPHC17/LConn2 -- CoolantCPHC18/LConn3 -- ThermalMassCPHC24/LConn1 -- TR_TMCPHC24/LConn1
  CoolantCPHC18/LConn2 -- CoolantCPHC19/LConn3 -- ThermalMassCPHC12/LConn1 -- TR_TMCPHC12/LConn1
  CoolantCPHC19/LConn2 -- CoolantCPHC20/LConn3 -- ThermalMassCPHC11/LConn1 -- TR_TMCPHC11/LConn1
  CoolantCPHC20/LConn2 -- CoolantCPHC21/LConn3 -- ThermalMassCPHC10/LConn1 -- TR_TMCPHC10/LConn1
  CoolantCPHC21/LConn2 -- CoolantCPHC31/LConn3 -- ThermalMassCPHC9/LConn1 -- TR_TMCPHC9/LConn1
  CoolantCPHC22/LConn3 -- ThermalMassCPHC13/LConn1 -- CoolantCPHC31/LConn2 -- TR_TMCPHC13/LConn1
  CoolantCPHC22/LConn2 -- CoolantCPHC23/LConn3 -- ThermalMassCPHC14/LConn1 -- TR_TMCPHC14/LConn1
  CoolantCPHC23/LConn2 -- CoolantCPHC24/LConn3 -- ThermalMassCPHC15/LConn1 -- TR_TMCPHC15/LConn1
  CoolantCPHC24/LConn2 -- CoolantCPHC25/LConn3 -- ThermalMassCPHC16/LConn1 -- TR_TMCPHC16/LConn1
  CoolantCPHC25/LConn2 -- CoolantCPHC26/LConn3 -- ThermalMassCPHC20/LConn1 -- TR_TMCPHC20/LConn1
  CoolantCPHC26/LConn2 -- CoolantCPHC27/LConn3 -- ThermalMassCPHC19/LConn1 -- TR_TMCPHC19/LConn1
  CoolantCPHC27/LConn2 -- CoolantCPHC28/LConn3 -- ThermalMassCPHC18/LConn1 -- TR_TMCPHC18/LConn1
  CoolantCPHC28/LConn2 -- CoolanthotCoolConnect63/LConn3 -- ThermalMassCPHC17/LConn1 -- TR_TMCPHC17/LConn1
  TR_TMCPCC1/RConn1 -- TR_TMCPHC1/RConn1 -- TR_MA1/RConn1 -- ThermalMassBatteries1/LConn1 -- heat1/LConn1
  TR_TMCPCC2/RConn1 -- TR_TMCPHC2/RConn1 -- TR_MA2/RConn1 -- ThermalMassBatteries2/LConn1 -- heat2/LConn1
  TR_TMCPCC3/RConn1 -- TR_TMCPHC3/RConn1 -- TR_MA3/RConn1 -- ThermalMassBatteries3/LConn1 -- heat3/LConn1
  TR_TMCPCC4/RConn1 -- TR_TMCPHC4/RConn1 -- TR_MA4/RConn1 -- ThermalMassBatteries4/LConn1 -- heat4/LConn1
  TR_TMCPCC5/RConn1 -- TR_TMCPHC5/RConn1 -- TR_MA5/RConn1 -- ThermalMassBatteries5/LConn1 -- heat5/LConn1
  TR_TMCPCC6/RConn1 -- TR_TMCPHC6/RConn1 -- TR_MA6/RConn1 -- ThermalMassBatteries6/LConn1 -- heat6/LConn1
  TR_TMCPCC7/RConn1 -- TR_TMCPHC7/RConn1 -- TR_MA7/RConn1 -- ThermalMassBatteries7/LConn1 -- heat7/LConn1
  TR_TMCPCC8/RConn1 -- TR_TMCPHC8/RConn1 -- TR_MA8/RConn1 -- ThermalMassBatteries8/LConn1 -- heat8/LConn1
  TR_TMCPCC9/RConn1 -- TR_TMCPHC9/RConn1 -- TR_MA9/RConn1 -- ThermalMassBatteries9/LConn1 -- heat9/LConn1
  TR_TMCPCC10/RConn1 -- TR_TMCPHC10/RConn1 -- TR_MA10/RConn1 -- ThermalMassBatteries10/LConn1 -- heat10/LConn1
  TR_TMCPCC11/RConn1 -- TR_TMCPHC11/RConn1 -- TR_MA11/RConn1 -- ThermalMassBatteries11/LConn1 -- heat11/LConn1
  TR_TMCPCC12/RConn1 -- TR_TMCPHC12/RConn1 -- TR_MA12/RConn1 -- ThermalMassBatteries12/LConn1 -- heat12/LConn1
  TR_TMCPCC13/RConn1 -- TR_TMCPHC13/RConn1 -- TR_MA13/RConn1 -- ThermalMassBatteries13/LConn1 -- heat13/LConn1
  TR_TMCPCC14/RConn1 -- TR_TMCPHC14/RConn1 -- TR_MA14/RConn1 -- ThermalMassBatteries14/LConn1 -- heat14/LConn1
  TR_TMCPCC15/RConn1 -- TR_TMCPHC15/RConn1 -- TR_MA15/RConn1 -- ThermalMassBatteries15/LConn1 -- heat15/LConn1
  TR_TMCPCC16/RConn1 -- TR_TMCPHC16/RConn1 -- TR_MA16/RConn1 -- ThermalMassBatteries16/LConn1 -- heat16/LConn1
  TR_TMCPCC17/RConn1 -- TR_TMCPHC17/RConn1 -- TR_MA17/RConn1 -- ThermalMassBatteries17/LConn1 -- heat17/LConn1
  TR_TMCPCC18/RConn1 -- TR_TMCPHC18/RConn1 -- TR_MA18/RConn1 -- ThermalMassBatteries18/LConn1 -- heat18/LConn1
  TR_TMCPCC19/RConn1 -- TR_TMCPHC19/RConn1 -- TR_MA19/RConn1 -- ThermalMassBatteries19/LConn1 -- heat19/LConn1
  TR_TMCPCC20/RConn1 -- TR_TMCPHC20/RConn1 -- TR_MA20/RConn1 -- ThermalMassBatteries20/LConn1 -- heat20/LConn1
  TR_TMCPCC21/RConn1 -- TR_TMCPHC21/RConn1 -- TR_MA21/RConn1 -- ThermalMassBatteries21/LConn1 -- heat21/LConn1
  TR_TMCPCC22/RConn1 -- TR_TMCPHC22/RConn1 -- TR_MA22/RConn1 -- ThermalMassBatteries22/LConn1 -- heat22/LConn1
  TR_TMCPCC23/RConn1 -- TR_TMCPHC23/RConn1 -- TR_MA23/RConn1 -- ThermalMassBatteries23/LConn1 -- heat23/LConn1
  TR_TMCPCC24/RConn1 -- TR_TMCPHC24/RConn1 -- TR_MA24/RConn1 -- ThermalMassBatteries24/LConn1 -- heat24/LConn1
  TR_TMCPCC25/RConn1 -- TR_TMCPHC25/RConn1 -- TR_MA25/RConn1 -- ThermalMassBatteries25/LConn1 -- heat25/LConn1
  TR_TMCPCC26/RConn1 -- TR_TMCPHC26/RConn1 -- TR_MA26/RConn1 -- ThermalMassBatteries26/LConn1 -- heat26/LConn1
  TR_TMCPCC27/RConn1 -- TR_TMCPHC27/RConn1 -- TR_MA27/RConn1 -- ThermalMassBatteries27/LConn1 -- heat27/LConn1
  TR_TMCPCC28/RConn1 -- TR_TMCPHC28/RConn1 -- TR_MA28/RConn1 -- ThermalMassBatteries28/LConn1 -- heat28/LConn1
  TR_TMCPCC29/RConn1 -- TR_TMCPHC29/RConn1 -- TR_MA29/RConn1 -- ThermalMassBatteries29/LConn1 -- heat29/LConn1
  TR_TMCPCC30/RConn1 -- TR_TMCPHC30/RConn1 -- TR_MA30/RConn1 -- ThermalMassBatteries30/LConn1 -- heat30/LConn1
  TR_TMCPCC31/RConn1 -- TR_TMCPHC31/RConn1 -- TR_MA31/RConn1 -- ThermalMassBatteries31/LConn1 -- heat31/LConn1
  TR_TMCPCC32/RConn1 -- TR_TMCPHC32/RConn1 -- TR_MA32/RConn1 -- ThermalMassBatteries32/LConn1 -- heat32/LConn1
  TempSource/RConn2 -- ThermalReference/LConn1 -- heat1/RConn2 -- heat2/RConn2 -- heat3/RConn2 -- heat4/RConn2 -- heat5/RConn2 -- heat6/RConn2 -- heat7/RConn2 -- heat8/RConn2 -- heat9/RConn2 -- heat10/RConn2 -- heat11/RConn2 -- heat12/RConn2 -- heat13/RConn2 -- heat14/RConn2 -- heat15/RConn2 -- heat16/RConn2 -- heat17/RConn2 -- heat18/RConn2 -- heat19/RConn2 -- heat20/RConn2 -- heat21/RConn2 -- heat22/RConn2 -- heat23/RConn2 -- heat24/RConn2 -- heat25/RConn2 -- heat26/RConn2 -- heat27/RConn2 -- heat28/RConn2 -- heat29/RConn2 -- heat30/RConn2 -- heat31/RConn2 -- heat32/RConn2 -- ThermalSolverConfig/RConn1
  ConstantTemp/RConn1 -- TempSource/RConn1
  TR_MA1/LConn1 -- TempSource/LConn1 -- TR_MA2/LConn1 -- TR_MA3/LConn1 -- TR_MA4/LConn1 -- TR_MA5/LConn1 -- TR_MA6/LConn1 -- TR_MA7/LConn1 -- TR_MA8/LConn1 -- TR_MA9/LConn1 -- TR_MA10/LConn1 -- TR_MA11/LConn1 -- TR_MA12/LConn1 -- TR_MA13/LConn1 -- TR_MA14/LConn1 -- TR_MA15/LConn1 -- TR_MA16/LConn1 -- TR_MA17/LConn1 -- TR_MA18/LConn1 -- TR_MA19/LConn1 -- TR_MA20/LConn1 -- TR_MA21/LConn1 -- TR_MA22/LConn1 -- TR_MA23/LConn1 -- TR_MA24/LConn1 -- TR_MA25/LConn1 -- TR_MA26/LConn1 -- TR_MA27/LConn1 -- TR_MA28/LConn1 -- TR_MA29/LConn1 -- TR_MA30/LConn1 -- TR_MA31/LConn1 -- TR_MA32/LConn1
  CoolantTempSource/LConn1 -- CoolantBC1/LConn2 -- CoolantBC2/LConn3
  SimulinkToPS1/RConn1 -- heat1/RConn1
  SimulinkToPS2/RConn1 -- heat2/RConn1
  SimulinkToPS3/RConn1 -- heat3/RConn1
  SimulinkToPS4/RConn1 -- heat4/RConn1
  SimulinkToPS5/RConn1 -- heat5/RConn1
  SimulinkToPS6/RConn1 -- heat6/RConn1
  SimulinkToPS7/RConn1 -- heat7/RConn1
  SimulinkToPS8/RConn1 -- heat8/RConn1
  SimulinkToPS9/RConn1 -- heat9/RConn1
  SimulinkToPS10/RConn1 -- heat10/RConn1
  SimulinkToPS11/RConn1 -- heat11/RConn1
  SimulinkToPS12/RConn1 -- heat12/RConn1
  SimulinkToPS13/RConn1 -- heat13/RConn1
  SimulinkToPS14/RConn1 -- heat14/RConn1
  SimulinkToPS15/RConn1 -- heat15/RConn1
  SimulinkToPS16/RConn1 -- heat16/RConn1
  SimulinkToPS17/RConn1 -- heat17/RConn1
  SimulinkToPS18/RConn1 -- heat18/RConn1
  SimulinkToPS19/RConn1 -- heat19/RConn1
  SimulinkToPS20/RConn1 -- heat20/RConn1
  SimulinkToPS21/RConn1 -- heat21/RConn1
  SimulinkToPS22/RConn1 -- heat22/RConn1
  SimulinkToPS23/RConn1 -- heat23/RConn1
  SimulinkToPS24/RConn1 -- heat24/RConn1
  SimulinkToPS25/RConn1 -- heat25/RConn1
  SimulinkToPS26/RConn1 -- heat26/RConn1
  SimulinkToPS27/RConn1 -- heat27/RConn1
  SimulinkToPS28/RConn1 -- heat28/RConn1
  SimulinkToPS29/RConn1 -- heat29/RConn1
  SimulinkToPS30/RConn1 -- heat30/RConn1
  SimulinkToPS31/RConn1 -- heat31/RConn1
  SimulinkToPS32/RConn1 -- heat32/RConn1
